simulink model "robot_model3"  (R2020b)
settings: Solver=ode4  StartTime=0.0  StopTime=50  FixedStep=T_s  RelTol=1e-3  EnableMultiTasking=on
InitFcn:
  | init_exp_icr
values from neighbouring files (symbols this model uses):
  D = [constd;constd;constd]    [init_exp_icr.m]
  g = 9.81    [init_exp_icr.m]
  K = [constx;consty;consttheta]    [init_exp_icr.m]
  l1 = 1    [init_exp_icr.m]
  lc1 = l1/2    (= 0.5)    [init_exp_icr.m]
  lc2 = l2/2    (= 0.5)    [init_exp_icr.m]
  m1 = 1    [init_exp_icr.m]
  m2 = 1    [init_exp_icr.m]
undefined symbols (not defined in the file or in its folder): I1zz, I2zz
settings Model: Creator=Lars  LastModifiedBy=jsol
settings SolverCC: AutoInsertRateTranBlk=on
settings DataIOCC: LimitDataPoints=on  SaveFormat=Array  ReturnWorkspaceOutputs=off
settings OptimizationCC: LifeSpan=inf
settings DebuggingCC: UnderspecifiedInitializationDetection=Classic  MergeDetectMultiDrivingBlocksExec=none  SolverPrmCheckMsg=warning  AllowSymbolicDim=off  SFUnexpectedBacktrackingDiag=warning  SFNoUnconditionalDefaultTransitionDiag=warning  SFExecutionAtInitializationDiag=none  ArithmeticOperatorsInVariantConditions=warning
settings HardwareCC: ProdBitPerPointer=32  ProdBitPerSizeT=32  ProdBitPerPtrDiffT=32  ProdLargestAtomicFloat=None  ProdIntDivRoundTo=Undefined  ProdEndianess=Unspecified  ProdWordSize=32  ProdHWDeviceType=32-bit Generic
settings ModelReferenceCC: PropagateSignalLabelsOutOfModel=off
settings SFSimCC: SimUseLocalCustomCode=off  CustomCodeUndefinedFunction=UseInterfaceOnly
settings RTWCC: RTWUseLocalCustomCode=off
settings CodeAppCC: StateflowObjectComments=on
settings GRTTargetCC: TargetLangStandard=C89/C90 (ANSI)
settings ConfigComp: CovMetricSettings=dw  CovSaveCumulativeToWorkspaceVar=on  CovSaveSingleToWorkspaceVar=on  CovExternalEMLEnable=off

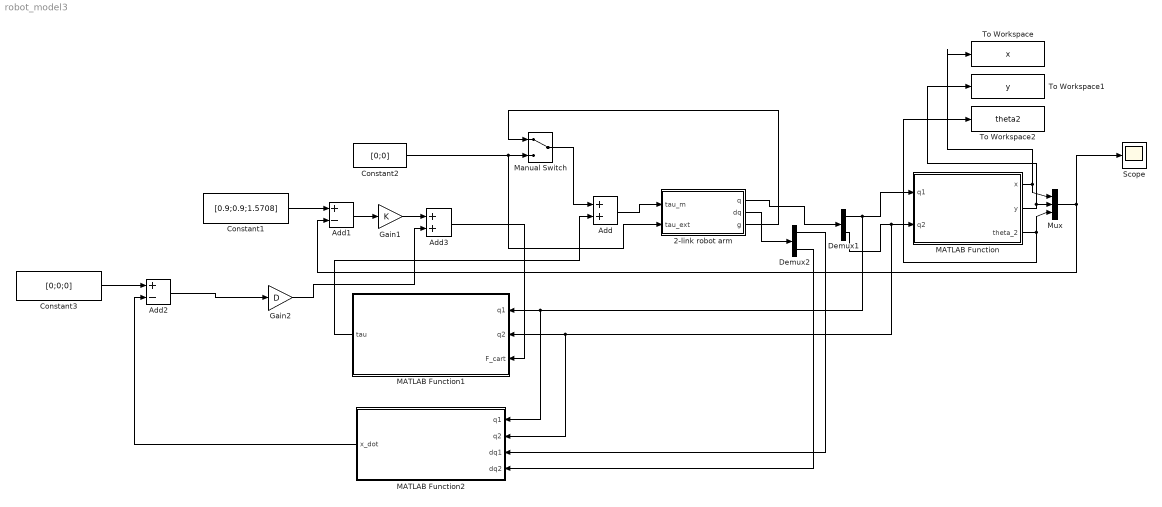
== system robot_model3 ==
  2-link robot arm : Subsystem
  Add : Sum
  Add1 : Sum  Inputs=+-
  Add2 : Sum  Inputs=+-
  Add3 : Sum
  Constant1 : Constant  Value=[0.9;0.9;1.5708]
  Constant2 : Constant  Value=[0;0]
  Constant3 : Constant  Value=[0;0;0]
  Demux1 : Demux  Outputs=2
  Demux2 : Demux  Outputs=2
  Gain1 : Gain  Gain=K
  Gain2 : Gain  Gain=D
  MATLAB Function : MATLAB Function  TreatAsAtomicUnit=on
  MATLAB Function1 : MATLAB Function  TreatAsAtomicUnit=on
  MATLAB Function2 : MATLAB Function  TreatAsAtomicUnit=on
  Manual Switch : ManualSwitch
  Mux : Mux  Inputs=3
  Scope : Scope
  To Workspace : ToWorkspace  VariableName=x  SaveFormat=Timeseries  SampleTime=-1
  To Workspace1 : ToWorkspace  VariableName=y  SaveFormat=Timeseries  SampleTime=-1
  To Workspace2 : ToWorkspace  VariableName=theta2  SaveFormat=Timeseries  SampleTime=-1
  wires:
  2-link robot arm/1("q ") -> Demux1/1
  MATLAB Function/1(x) -> To Workspace/1, Mux/1
  Add/1 -> 2-link robot arm/1(tau_m)
  2-link robot arm/3(g) -> Manual Switch/1
  Manual Switch/1 -> Add/1
  Constant1/1 -> Add1/1
  Add1/1 -> Gain1/1
  Constant2/1 -> Manual Switch/2, 2-link robot arm/2(tau_ext)
  Demux1/1 -> MATLAB Function2/1(q1), MATLAB Function1/1(q1), MATLAB Function/1(q1)
  Demux1/2 -> MATLAB Function2/2(q2), MATLAB Function1/2(q2), MATLAB Function/2(q2)
  MATLAB Function/2(y) -> To Workspace1/1, Mux/2
  MATLAB Function/3(theta_2) -> To Workspace2/1, Mux/3
  Mux/1 -> Scope/1, Add1/2
  MATLAB Function1/1(tau) -> Add/2
  2-link robot arm/2("dq ") -> Demux2/1
  Demux2/1 -> MATLAB Function2/3(dq1)
  Demux2/2 -> MATLAB Function2/4(dq2)
  Constant3/1 -> Add2/1
  MATLAB Function2/1(x_dot) -> Add2/2
  Add2/1 -> Gain2/1
  Gain1/1 -> Add3/1
  Add3/1 -> MATLAB Function1/3(F_cart)
  Gain2/1 -> Add3/2

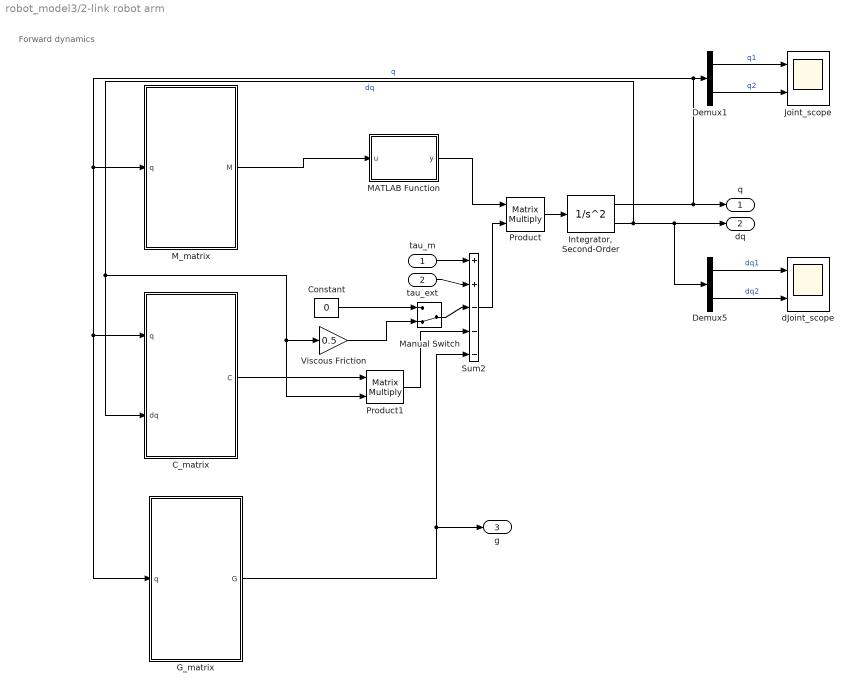
== system robot_model3/2-link robot arm ==
  note: Forward dynamics
  tau_m : Inport
  tau_ext : Inport  Port=2
  C_matrix : MATLAB Function  TreatAsAtomicUnit=on
  Constant : Constant  Value=0
  Demux1 : Demux  Outputs=2
  Demux5 : Demux  Outputs=2
  G_matrix : MATLAB Function  TreatAsAtomicUnit=on
  "Integrator, Second-Order" : SecondOrderIntegrator  ICX=[0,0]  ICDXDT=[0 0]
  Joint_scope : Scope  NumInputPorts=2
  MATLAB Function : MATLAB Function  TreatAsAtomicUnit=on
  M_matrix : MATLAB Function  TreatAsAtomicUnit=on
  Manual Switch : ManualSwitch  CurrentSetting=0
  Product : Product  Multiplication=Matrix(*)
  Product1 : Product  Multiplication=Matrix(*)
  Sum2 : Sum  Inputs=++|---
  Viscous Friction : Gain  Gain=0.5
  dJoint_scope : Scope  NumInputPorts=2
  "q " : Outport
  "dq " : Outport  Port=2
  g : Outport  Port=3
  wires:
  Demux1/1 -> Joint_scope/1  "q1"
  Demux1/2 -> Joint_scope/2  "q2"
  "Integrator, Second-Order"/2 -> Demux5/1, "dq "/1, Product1/2, Viscous Friction/1, C_matrix/2(dq)  "dq"
  Demux5/1 -> dJoint_scope/1  "dq1"
  C_matrix/1(C) -> Product1/1
  "Integrator, Second-Order"/1 -> "q "/1, Demux1/1, G_matrix/1(q), C_matrix/1(q), M_matrix/1(q)  "q"
  Demux5/2 -> dJoint_scope/2  "dq2"
  Sum2/1 -> Product/2
  Constant/1 -> Manual Switch/1
  Viscous Friction/1 -> Manual Switch/2
  M_matrix/1(M) -> MATLAB Function/1(u)
  Product/1 -> "Integrator, Second-Order"/1
  G_matrix/1(G) -> Sum2/5, g/1
  Product1/1 -> Sum2/4
  Manual Switch/1 -> Sum2/3
  tau_m/1 -> Sum2/1
  tau_ext/1 -> Sum2/2
  MATLAB Function/1(y) -> Product/1

== matlab function robot_model3/2-link robot arm/C_matrix ==
  data: q input; C output; dq input; l1 parameter; lc2 parameter; m2 parameter
function C = C_matrix(q,dq, l1, lc2, m2)
%#codegen

%    This function was generated by the Symbolic Math Toolbox version 8.3.
%    05-Nov-2019 15:18:30
q1 = q(1);
q2 = q(2);
dq1 = dq(1);
dq2 = dq(2);
t2 = sin(q2);
C = reshape([-dq2.*l1.*lc2.*m2.*t2,dq1.*l1.*lc2.*m2.*t2,-l1.*lc2.*m2.*t2.*(dq1+dq2),0.0],[2,2]);

== matlab function robot_model3/2-link robot arm/M_matrix ==
  data: M output; q input; I1zz parameter; I2zz parameter; l1 parameter; lc1 parameter; lc2 parameter; m1 parameter; m2 parameter
function M = M_matrix(q, I1zz, I2zz, l1, lc1, lc2, m1, m2)
%#codegen

%    This function was generated by the Symbolic Math Toolbox version 8.3.
%    05-Nov-2019 15:18:29
q1 = q(1);
q2 = q(2);
t2 = cos(q2);
t3 = lc2.^2;
t4 = m2.*t3;
t5 = l1.*lc2.*m2.*t2;
t6 = I2zz+t4+t5;
M = reshape([I1zz+t5+t6+l1.^2.*m2+lc1.^2.*m1,t6,t6,I2zz+t4],[2,2]);

== matlab function robot_model3/2-link robot arm/MATLAB Function ==
  data: u input; y output
function y = inverse_matrix(u)
    if det(u) ~= 0
        y = inv(u);
    else
        y = zeros(size(u)); % or handle singular case differently
    end
end

== matlab function robot_model3/MATLAB Function ==
  data: x output; q1 input; y output; q2 input; theta_2 output
function [x, y, theta_2] = directKinematics(q1, q2)
%#codegen
% Inputs:
%   q1, q2 - joint angles [rad]
%   l1, l2 - link lengths
% Outputs:
%   x, y - end-effector Cartesian position
%   theta_ee - end-effector orientation angle

% Position of end-effector
x =  cos(q1) +  cos(q1 + q2);
y =  sin(q1) +  sin(q1 + q2);

% Orientation (absolute)
theta_2 = q1 + q2;
end

== matlab function robot_model3/MATLAB Function1 ==
  data: q1 input; tau output; q2 input; F_cart input
function tau = jacobianForceMap(q1, q2, F_cart)
%#codegen
% Inputs:
%   q1, q2   - joint angles [rad]
%   F_cart   - 3x1 Cartesian force/torque vector [Fx; Fy; Tz]
% Output:
%   tau      - 2x1 joint torques

% Precompute trigonometric terms
s1 = sin(q1);
s12 = sin(q1 + q2);
c1 = cos(q1);
c12 = cos(q1 + q2);

% Compute Jacobian transpose (2x3)
J_T = [ -s1 - s12,  c1 + c12,  1;
        -s12,       c12,       1 ];

% Multiply by Cartesian force to get joint torques
tau = J_T * F_cart;
end

== matlab function robot_model3/MATLAB Function2 ==
  data: q1 input; x_dot output; q2 input; dq1 input; dq2 input
function x_dot = cartesianVelocity(q1, q2, dq1, dq2)
%#codegen

s1 = sin(q1); s12 = sin(q1 + q2);
c1 = cos(q1); c12 = cos(q1 + q2);

J = [ -s1 - s12, -s12;
       c1 + c12,  c12;
       1,         1 ];

% Joint velocity vector
dq = [dq1; dq2];

% Cartesian velocity
x_dot = J * dq;
end

== matlab function robot_model3/2-link robot arm/G_matrix ==
  data: G output; q input; g parameter; l1 parameter; lc1 parameter; lc2 parameter; m1 parameter; m2 parameter
function G = G_matrix(q, g, l1, lc1, lc2, m1, m2)
%#codegen

%    This function was generated by the Symbolic Math Toolbox version 8.3.
%    05-Nov-2019 15:18:30
q1 = q(1);
q2 = q(2);
t2 = cos(q1);
t3 = q1+q2;
t4 = cos(t3);
G = [g.*m2.*(l1.*t2+lc2.*t4)+g.*lc1.*m1.*t2;g.*lc2.*m2.*t4];
